simulink model "mitchell_bluetooth"  (R2018b)
settings: Solver=FixedStepDiscrete  StartTime=0.0  StopTime=10.0  FixedStep=0.00005  RelTol=1e-3  EnableMultiTasking=on
libraries: stellaris_lp_lib x13, discretizing x3, etargetslib x1, xpcutilitieslib x1
settings Model: Creator=Mitchell Cassaday  LastModifiedBy=Mitchell Cassaday
settings OptimizationCC: DefaultUnderspecifiedDataType=single  PassReuseOutputArgsAs=Individual arguments  MaxStackSize=64
settings DebuggingCC: BlockPriorityViolationMsg=error  MinStepSizeMsg=error  SolverPrmCheckMsg=warning  MultiTaskRateTransMsg=warning  ParameterTunabilityLossMsg=error
settings HardwareCC: ProdBitPerPointer=32  ProdBitPerSizeT=32  ProdBitPerPtrDiffT=32  ProdLargestAtomicInteger=Long  ProdLargestAtomicFloat=Double  ProdWordSize=32  ProdHWDeviceType=ARM Compatible->ARM Cortex
settings SFSimCC: SimUseLocalCustomCode=off  MATLABDynamicMemAlloc=off
settings RTWCC: SystemTargetFile=ert.tlc  HardwareBoard=Tiva TM4C123G Launchpad  TemplateMakefile=ert_default_tmf  GenerateReport=on  RTWUseLocalCustomCode=off  Toolchain=Texas Instruments Code Composer Studio (Tiva)  BuildConfiguration=Faster Runs  IncludeHyperlinkInReport=on  LaunchReport=on  GenerateTraceInfo=on  GenerateTraceReport=on  GenerateTraceReportSl=on  GenerateTraceReportSf=on  GenerateTraceReportEml=on
settings CodeAppCC: ForceParamTrailComments=on  IgnoreCustomStorageClasses=off  OperatorAnnotations=on  SimulinkDataObjDesc=on  SFDataObjDesc=on  InsertBlockDesc=on

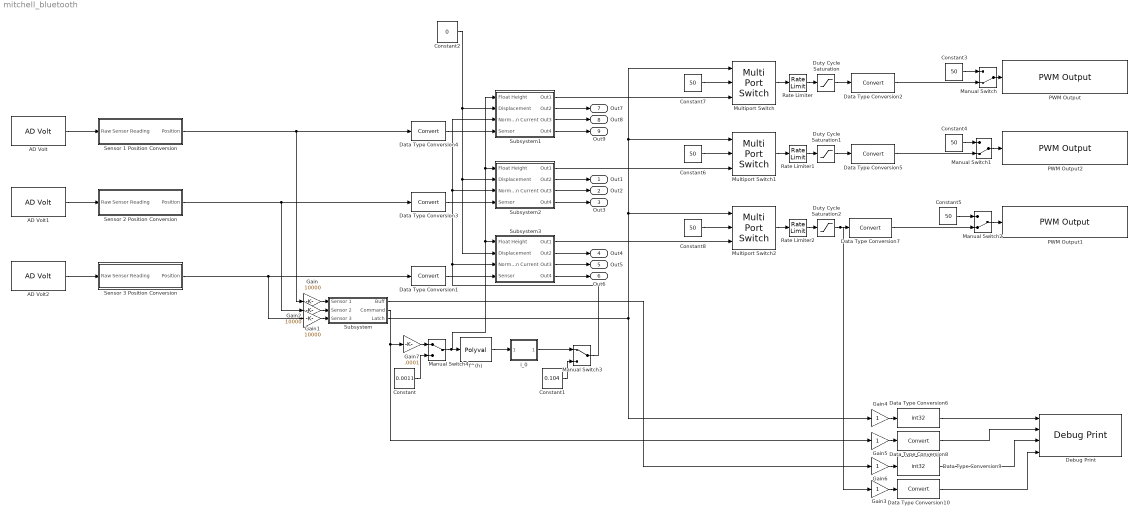
== system mitchell_bluetooth ==
  AD Volt : stellaris_lp_lib/ADC/AD Volt  ch="5   PE5"  sample_time=0.0001
      settings: SourceProductName=Run on Stellaris LaunchPad
  AD Volt1 : stellaris_lp_lib/ADC/AD Volt  ch="3   PE1"  sample_time=0.0001
      settings: SourceProductName=Run on Stellaris LaunchPad
  AD Volt2 : stellaris_lp_lib/ADC/AD Volt  ch="2   PE2"  sample_time=0.0001
      settings: SourceProductName=Run on Stellaris LaunchPad
  Constant : Constant  Value=0.0011
  Constant1 : Constant  Value=0.104
  Constant2 : Constant  Value=0
  Constant{3..8} (6 alike) : Constant  Value=50
  Data Type Conversion{1..5,7..8,10} (8 alike) : DataTypeConversion
  Data Type Conversion6 : DataTypeConversion  OutDataTypeStr=int32
  Data Type Conversion9 : DataTypeConversion  OutDataTypeStr=int32
  Debug Print : stellaris_lp_lib/Debug/Debug Print  fmt="'a: %d    b: %d    c: %d     d:%d'"  sample_time=0.1
      settings: SourceProductName=Run on Stellaris LaunchPad
  Duty Cycle Saturation : Saturate  UpperLimit=99  LowerLimit=0
  Duty Cycle Saturation1 : Saturate  UpperLimit=99  LowerLimit=0
  Duty Cycle Saturation2 : Saturate  UpperLimit=99  LowerLimit=0
  Gain : Gain  Gain=10000
  Gain1 : Gain  Gain=10000
  Gain2 : Gain  Gain=10000
  Gain{3..6} (4 alike) : Gain
  Gain7 : Gain  Gain=.0001
  Manual Switch : ManualSwitch  CurrentSetting=0
  Manual Switch1 : ManualSwitch  CurrentSetting=0
  Manual Switch2 : ManualSwitch  CurrentSetting=0
  Manual Switch3 : ManualSwitch
  Manual Switch4 : ManualSwitch
  Multiport Switch : MultiPortSwitch  DataPortOrder=Zero-based contiguous  Inputs=2  DiagnosticForDefault=None  zeroidx=on
  Multiport Switch1 : MultiPortSwitch  DataPortOrder=Zero-based contiguous  Inputs=2  DiagnosticForDefault=None  zeroidx=on
  Multiport Switch2 : MultiPortSwitch  DataPortOrder=Zero-based contiguous  Inputs=2  DiagnosticForDefault=None  zeroidx=on
  PWM Output : stellaris_lp_lib/PWM/PWM Output  ch="1    PC4"  invert=off  freq=100000  sample_time=-1
      settings: SourceProductName=Run on Stellaris LaunchPad
  PWM Output1 : stellaris_lp_lib/PWM/PWM Output  ch="3    PC6"  invert=off  freq=100000  sample_time=-1
      settings: SourceProductName=Run on Stellaris LaunchPad
  PWM Output2 : stellaris_lp_lib/PWM/PWM Output  ch="2    PC5"  invert=off  freq=100000  sample_time=-1
      settings: SourceProductName=Run on Stellaris LaunchPad
  Rate Limiter : RateLimiter  RisingSlewLimit=10000  FallingSlewLimit=-10000  SampleTimeMode=inherited
  Rate Limiter1 : RateLimiter  RisingSlewLimit=10000  FallingSlewLimit=-10000  SampleTimeMode=inherited
  Rate Limiter2 : RateLimiter  RisingSlewLimit=10000  FallingSlewLimit=-10000  SampleTimeMode=inherited
  Sensor 1 Position Conversion : Subsystem
  Sensor 2 Position Conversion : Subsystem
  Sensor 3 Position Conversion : Subsystem
  Subsystem : Subsystem
  Subsystem1 : Subsystem
  Subsystem2 : Subsystem
  Subsystem3 : Subsystem
  f^(h) : Polyval  Coefs=[ +1.6739e+20, -1.3935e+18, +4.7154e+15, -8.351e+12, +8.2878e+9, -4.527e+6, 1.1593e+3 ]
  "i_0 " : Subsystem
  Out1 : Outport
  Out2 : Outport  Port=2
  Out3 : Outport  Port=3
  Out4 : Outport  Port=4
  Out5 : Outport  Port=5
  Out6 : Outport  Port=6
  Out7 : Outport  Port=7
  Out8 : Outport  Port=8
  Out9 : Outport  Port=9
  wires:
  AD Volt2/1 -> Sensor 3 Position Conversion/1(Raw Sensor Reading)
  AD Volt1/1 -> Sensor 2 Position Conversion/1(Raw Sensor Reading)
  AD Volt/1 -> Sensor 1 Position Conversion/1(Raw Sensor Reading)
  Data Type Conversion3/1 -> Subsystem2/4(Sensor)
  Data Type Conversion4/1 -> Subsystem1/4(Sensor)
  Constant2/1 -> Subsystem1/2(Displacement), Subsystem3/2(Displacement), Subsystem2/2(Displacement)
  Manual Switch3/1 -> Subsystem1/3(Normalization Current), Subsystem2/3(Normalization Current), Subsystem3/3(Normalization Current)
  Manual Switch2/1 -> PWM Output1/1
  Manual Switch1/1 -> PWM Output2/1
  Subsystem2/4(Out4) -> Out3/1
  Data Type Conversion6/1 -> Debug Print/1
  Manual Switch/1 -> PWM Output/1
  Data Type Conversion2/1 -> Manual Switch/2
  Constant3/1 -> Manual Switch/1
  Data Type Conversion5/1 -> Manual Switch1/2
  Constant4/1 -> Manual Switch1/1
  Data Type Conversion7/1 -> Manual Switch2/2
  Constant5/1 -> Manual Switch2/1
  Data Type Conversion8/1 -> Debug Print/2
  Data Type Conversion9/1 -> Debug Print/3
  Data Type Conversion10/1 -> Debug Print/4
  Subsystem2/2(Out2) -> Out1/1
  Subsystem2/3(Out3) -> Out2/1
  Subsystem3/3(Out3) -> Out5/1
  Subsystem3/2(Out2) -> Out4/1
  Subsystem3/4(Out4) -> Out6/1
  Subsystem1/4(Out4) -> Out9/1
  Subsystem1/2(Out2) -> Out7/1
  Subsystem1/3(Out3) -> Out8/1
  Data Type Conversion1/1 -> Subsystem3/4(Sensor)
  Sensor 1 Position Conversion/1(Position) -> Data Type Conversion4/1, Gain/1
  Sensor 2 Position Conversion/1(Position) -> Data Type Conversion3/1, Gain1/1
  Gain/1 -> Subsystem/1("Sensor 1 ")
  Gain1/1 -> Subsystem/2(Sensor 2)
  Gain3/1 -> Data Type Conversion10/1
  Gain2/1 -> Subsystem/3(Sensor 3)
  Gain4/1 -> Data Type Conversion6/1
  Gain5/1 -> Data Type Conversion8/1
  Gain6/1 -> Data Type Conversion9/1
  Sensor 3 Position Conversion/1(Position) -> Data Type Conversion1/1, Gain2/1
  f^(h)/1 -> "i_0 "/1(f^(h0))
  Constant/1 -> Manual Switch4/2
  Constant1/1 -> Manual Switch3/2
  "i_0 "/1(Out1) -> Manual Switch3/1
  Subsystem/1(Buff) -> Gain6/1
  Subsystem1/1(Out1) -> Multiport Switch/3
  Subsystem3/1(Out1) -> Multiport Switch2/3
  Duty Cycle Saturation/1 -> Data Type Conversion2/1
  Duty Cycle Saturation1/1 -> Data Type Conversion5/1
  Duty Cycle Saturation2/1 -> Gain3/1, Data Type Conversion7/1
  Subsystem/2(Command) -> Gain5/1, Gain7/1
  Gain7/1 -> Manual Switch4/1
  Manual Switch4/1 -> f^(h)/1, Subsystem3/1(Float Height), Subsystem2/1(Float Height), Subsystem1/1(Float Height)
  Subsystem/3("Latch ") -> Gain4/1, Multiport Switch/1, Multiport Switch1/1, Multiport Switch2/1
  Multiport Switch/1 -> Rate Limiter/1
  Rate Limiter/1 -> Duty Cycle Saturation/1
  Multiport Switch1/1 -> Rate Limiter1/1
  Rate Limiter1/1 -> Duty Cycle Saturation1/1
  Multiport Switch2/1 -> Rate Limiter2/1
  Rate Limiter2/1 -> Duty Cycle Saturation2/1
  Subsystem2/1(Out1) -> Multiport Switch1/3
  Constant6/1 -> Multiport Switch1/2
  Constant7/1 -> Multiport Switch/2
  Constant8/1 -> Multiport Switch2/2

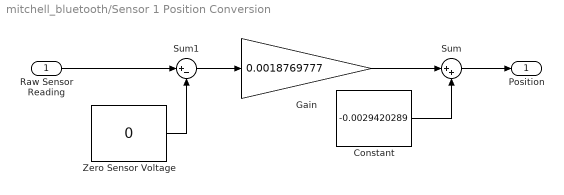
== system mitchell_bluetooth/Sensor 1 Position Conversion ==
  Raw Sensor Reading : Inport
  Constant : Constant  Value=-0.0029420289  OutDataTypeStr=Inherit: Inherit via back propagation
  Gain : Gain  Gain=0.0018769777
  Sum : Sum  Inputs=|++
  Sum1 : Sum  Inputs=|+-
  Zero Sensor Voltage : Constant  Value=0  OutDataTypeStr=Inherit: Inherit via back propagation
  Position : Outport
  wires:
  Gain/1 -> Sum/1
  Constant/1 -> Sum/2
  Sum/1 -> Position/1
  Zero Sensor Voltage/1 -> Sum1/2
  Sum1/1 -> Gain/1
  Raw Sensor Reading/1 -> Sum1/1

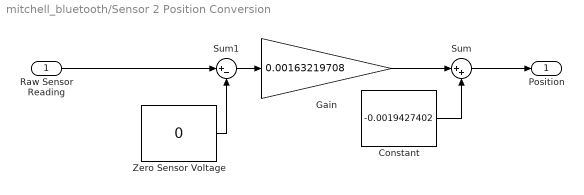
== system mitchell_bluetooth/Sensor 2 Position Conversion ==
  Raw Sensor Reading : Inport
  Constant : Constant  Value=-0.0019427402  OutDataTypeStr=Inherit: Inherit via back propagation
  Gain : Gain  Gain=0.00163219708
  Sum : Sum  Inputs=|++
  Sum1 : Sum  Inputs=|+-
  Zero Sensor Voltage : Constant  Value=0  OutDataTypeStr=Inherit: Inherit via back propagation
  Position : Outport
  wires:
  Gain/1 -> Sum/1
  Constant/1 -> Sum/2
  Sum/1 -> Position/1
  Zero Sensor Voltage/1 -> Sum1/2
  Sum1/1 -> Gain/1
  Raw Sensor Reading/1 -> Sum1/1

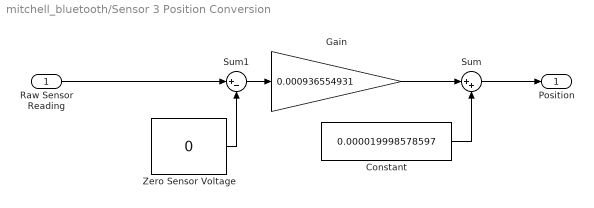
== system mitchell_bluetooth/Sensor 3 Position Conversion ==
  Raw Sensor Reading : Inport
  Constant : Constant  Value=0.000019998578597  OutDataTypeStr=Inherit: Inherit via back propagation
  Gain : Gain  Gain=0.000936554931
  Sum : Sum  Inputs=|++
  Sum1 : Sum  Inputs=|+-
  Zero Sensor Voltage : Constant  Value=0  OutDataTypeStr=Inherit: Inherit via back propagation
  Position : Outport
  wires:
  Gain/1 -> Sum/1
  Constant/1 -> Sum/2
  Sum/1 -> Position/1
  Zero Sensor Voltage/1 -> Sum1/2
  Sum1/1 -> Gain/1
  Raw Sensor Reading/1 -> Sum1/1

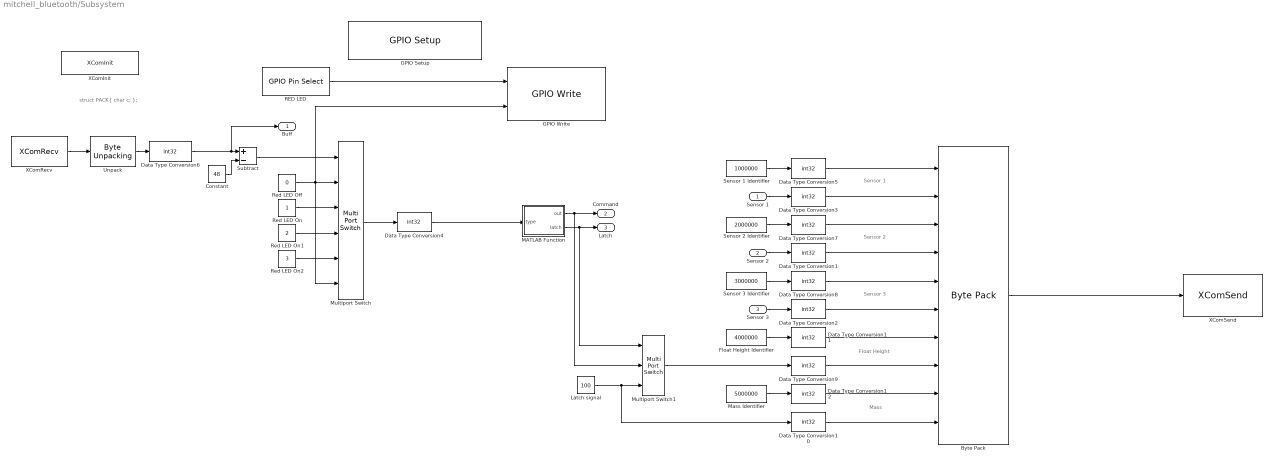
== system mitchell_bluetooth/Subsystem ==
  note: Sensor 1
  note: struct  PACK{
      | 		char c;
      | };
  note: Sensor 2
  note: Sensor 3
  note: Float Height
  note: Mass
  "Sensor 1 " : Inport
  Sensor 2 : Inport  Port=2
  Sensor 3 : Inport  Port=3
  Byte Pack : etargetslib/Byte Pack  datatypes={'int32','int32','int32','int32','int32','int32','int32','int32','int32','int32'}  byteAlign=1
  Constant : Constant  Value=48  OutDataTypeStr=int32
  Data Type Conversion{1..12} (12 alike) : DataTypeConversion  OutDataTypeStr=int32
  Float Height Identifier : Constant  Value=4000000  OutDataTypeStr=int32
  GPIO Setup : stellaris_lp_lib/GPIO/GPIO Setup  GPIO_PORTX_BASE=GPIO_PORTF_BASE  PinsOutput_0=Input  PinsOutput_1=Output  PinsOutput_2=Output  PinsOutput_3=Output  PinsOutput_4=Input  PinsOutput_5=Input  PinsOutput_6=Input  PinsOutput_7=Input
      settings: SourceProductName=Run on Stellaris LaunchPad
  GPIO Write : stellaris_lp_lib/GPIO/GPIO Write  GPIO_PORTX_BASE=GPIO_PORTF_BASE  SampleTime=-1
      settings: SourceProductName=Run on Stellaris LaunchPad
  Latch signal : Constant  Value=100  OutDataTypeStr=uint8
  MATLAB Function : MATLAB Function  TreatAsAtomicUnit=on
  Mass Identifier : Constant  Value=5000000  OutDataTypeStr=int32
  Multiport Switch : MultiPortSwitch  DataPortOrder=Zero-based contiguous  Inputs=5  DiagnosticForDefault=None  zeroidx=on
  Multiport Switch1 : MultiPortSwitch  DataPortOrder=Zero-based contiguous  Inputs=2  DiagnosticForDefault=None  zeroidx=on
  RED LED : stellaris_lp_lib/GPIO/GPIO Pin Select  GPIO_PIN_X=GPIO_PIN_1
      settings: SourceProductName=Run on Stellaris LaunchPad
  Red LED Off : Constant  Value=0  OutDataTypeStr=uint8
  Red LED On : Constant  OutDataTypeStr=uint8
  Red LED On1 : Constant  Value=2  OutDataTypeStr=uint8
  Red LED On2 : Constant  Value=3  OutDataTypeStr=uint8
  Sensor 1 Identifier : Constant  Value=1000000  OutDataTypeStr=int32
  Sensor 2 Identifier : Constant  Value=2000000  OutDataTypeStr=int32
  Sensor 3 Identifier : Constant  Value=3000000  OutDataTypeStr=int32
  Subtract : Sum  Inputs=+-
  Unpack : xpcutilitieslib/Byte Unpacking   MaskUnpackedDataTypes={'uint8'}  MaskUnpackedDataSizes={1}  MaskAlignment=1
      settings: SourceProductName=Simulink Real-Time  SourceProductBaseCode=XP
  XComInit : stellaris_lp_lib/Communication/XComInit  baud=9600
      settings: SourceProductName=Run on Stellaris LaunchPad
  XComRecv : stellaris_lp_lib/Communication/XComRecv  pack_size=1  sample_time=.001
      settings: SourceProductName=Run on Stellaris LaunchPad
  XComSend : stellaris_lp_lib/Communication/XComSend  pack_size=40  sample_time=0.1
      settings: SourceProductName=Run on Stellaris LaunchPad
  Buff : Outport
  Command : Outport  Port=2
  "Latch " : Outport  Port=3
  wires:
  XComRecv/1 -> Unpack/1
  Unpack/1 -> Data Type Conversion6/1
  Byte Pack/1 -> XComSend/1
  Red LED On/1 -> Multiport Switch/3
  "Sensor 1 "/1 -> Data Type Conversion3/1
  Constant/1 -> Subtract/2
  Red LED Off/1 -> Multiport Switch/6, GPIO Write/2, Multiport Switch/2
  RED LED/1 -> GPIO Write/1
  Sensor 2/1 -> Data Type Conversion1/1
  Sensor 3/1 -> Data Type Conversion2/1
  MATLAB Function/1(out) -> Command/1, Multiport Switch1/2
  Subtract/1 -> Multiport Switch/1
  Multiport Switch/1 -> Data Type Conversion4/1
  Red LED On1/1 -> Multiport Switch/4
  Red LED On2/1 -> Multiport Switch/5
  Data Type Conversion4/1 -> MATLAB Function/1(type)
  MATLAB Function/2(latch) -> Multiport Switch1/1, "Latch "/1
  Data Type Conversion6/1 -> Subtract/1, Buff/1
  Sensor 1 Identifier/1 -> Data Type Conversion5/1
  Data Type Conversion1/1 -> Byte Pack/4
  Sensor 2 Identifier/1 -> Data Type Conversion7/1
  Data Type Conversion3/1 -> Byte Pack/2
  Sensor 3 Identifier/1 -> Data Type Conversion8/1
  Data Type Conversion2/1 -> Byte Pack/6
  Data Type Conversion5/1 -> Byte Pack/1
  Data Type Conversion7/1 -> Byte Pack/3
  Data Type Conversion8/1 -> Byte Pack/5
  Data Type Conversion11/1 -> Byte Pack/7
  Data Type Conversion9/1 -> Byte Pack/8
  Data Type Conversion12/1 -> Byte Pack/9
  Data Type Conversion10/1 -> Byte Pack/10
  Float Height Identifier/1 -> Data Type Conversion11/1
  Mass Identifier/1 -> Data Type Conversion12/1
  Latch signal/1 -> Data Type Conversion10/1, Multiport Switch1/3
  Multiport Switch1/1 -> Data Type Conversion9/1

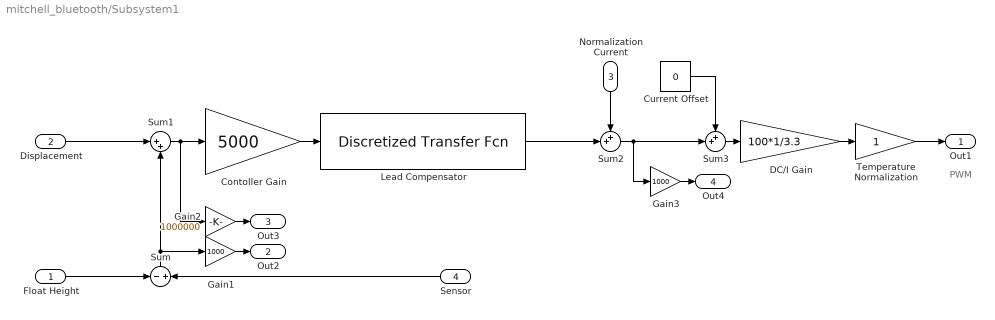
== system mitchell_bluetooth/Subsystem1 ==
  note: PWM
  Float Height : Inport
  Displacement : Inport  Port=2
  Normalization Current : Inport  Port=3
  Sensor : Inport  Port=4
  Contoller Gain : Gain  Gain=5000
  Current Offset : Constant  Value=0
  DC/I Gain : Gain  Gain=100*1/3.3
  Gain1 : Gain  Gain=1000
  Gain2 : Gain  Gain=1000000
  Gain3 : Gain  Gain=1000
  Lead Compensator : discretizing/Discretized Transfer Fcn  Numerator=[1 550]  Denominator=[1 3100]  AbsTol=auto  SampleTime=0.0001  method=zoh  Wc=0
  Sum : Sum  Inputs=-|+
  Sum1 : Sum  Inputs=|++
  Sum2 : Sum  Inputs=++|
  Sum3 : Sum  Inputs=++|
  Temperature Normalization : Gain
  Out1 : Outport  OutMin=[0]  OutMax=[100]
  Out2 : Outport  Port=2
  Out3 : Outport  Port=3
  Out4 : Outport  Port=4
  wires:
  Gain3/1 -> Out4/1
  Sum/1 -> Gain1/1, Sum1/2
  Contoller Gain/1 -> Lead Compensator/1
  Lead Compensator/1 -> Sum2/2
  Sum2/1 -> Sum3/2, Gain3/1
  Gain1/1 -> Out2/1
  Float Height/1 -> Sum/1
  Temperature Normalization/1 -> Out1/1
  Gain2/1 -> Out3/1
  Sensor/1 -> Sum/2
  Sum1/1 -> Gain2/1, Contoller Gain/1
  Displacement/1 -> Sum1/1
  Normalization Current/1 -> Sum2/1
  Sum3/1 -> DC/I Gain/1
  DC/I Gain/1 -> Temperature Normalization/1
  Current Offset/1 -> Sum3/1

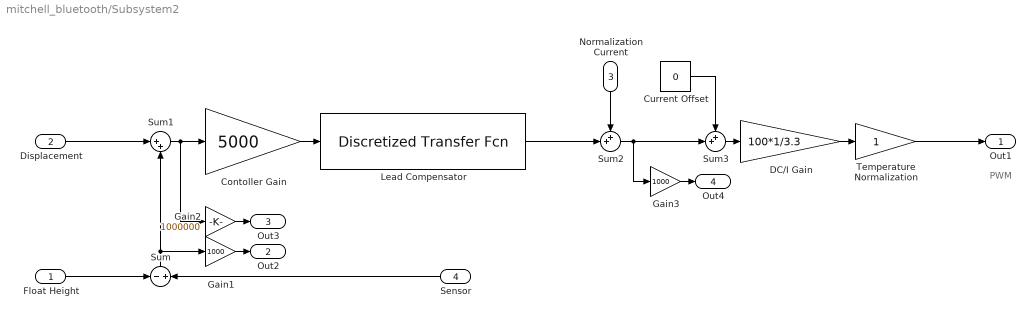
== system mitchell_bluetooth/Subsystem2 ==
  note: PWM
  Float Height : Inport
  Displacement : Inport  Port=2
  Normalization Current : Inport  Port=3
  Sensor : Inport  Port=4
  Contoller Gain : Gain  Gain=5000
  Current Offset : Constant  Value=0
  DC/I Gain : Gain  Gain=100*1/3.3
  Gain1 : Gain  Gain=1000
  Gain2 : Gain  Gain=1000000
  Gain3 : Gain  Gain=1000
  Lead Compensator : discretizing/Discretized Transfer Fcn  Numerator=[1 550]  Denominator=[1 3100]  AbsTol=auto  SampleTime=0.0001  method=zoh  Wc=0
  Sum : Sum  Inputs=-|+
  Sum1 : Sum  Inputs=|++
  Sum2 : Sum  Inputs=++|
  Sum3 : Sum  Inputs=++|
  Temperature Normalization : Gain
  Out1 : Outport  OutMin=[0]  OutMax=[100]
  Out2 : Outport  Port=2
  Out3 : Outport  Port=3
  Out4 : Outport  Port=4
  wires:
  Gain3/1 -> Out4/1
  Sum/1 -> Gain1/1, Sum1/2
  Contoller Gain/1 -> Lead Compensator/1
  Lead Compensator/1 -> Sum2/2
  Sum2/1 -> Sum3/2, Gain3/1
  Gain1/1 -> Out2/1
  Float Height/1 -> Sum/1
  Temperature Normalization/1 -> Out1/1
  Gain2/1 -> Out3/1
  Sensor/1 -> Sum/2
  Sum1/1 -> Gain2/1, Contoller Gain/1
  Displacement/1 -> Sum1/1
  Normalization Current/1 -> Sum2/1
  Sum3/1 -> DC/I Gain/1
  DC/I Gain/1 -> Temperature Normalization/1
  Current Offset/1 -> Sum3/1

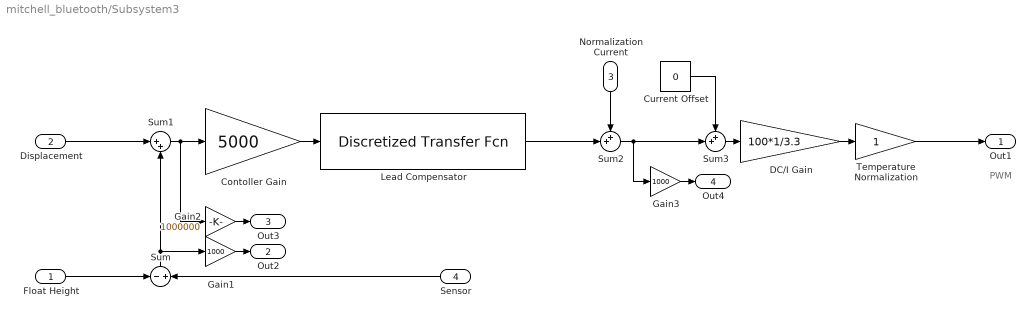
== system mitchell_bluetooth/Subsystem3 ==
  note: PWM
  Float Height : Inport
  Displacement : Inport  Port=2
  Normalization Current : Inport  Port=3
  Sensor : Inport  Port=4
  Contoller Gain : Gain  Gain=5000
  Current Offset : Constant  Value=0
  DC/I Gain : Gain  Gain=100*1/3.3
  Gain1 : Gain  Gain=1000
  Gain2 : Gain  Gain=1000000
  Gain3 : Gain  Gain=1000
  Lead Compensator : discretizing/Discretized Transfer Fcn  Numerator=[1 550]  Denominator=[1 3100]  AbsTol=auto  SampleTime=0.0001  method=zoh  Wc=0
  Sum : Sum  Inputs=-|+
  Sum1 : Sum  Inputs=|++
  Sum2 : Sum  Inputs=++|
  Sum3 : Sum  Inputs=++|
  Temperature Normalization : Gain
  Out1 : Outport  OutMin=[0]  OutMax=[100]
  Out2 : Outport  Port=2
  Out3 : Outport  Port=3
  Out4 : Outport  Port=4
  wires:
  Gain3/1 -> Out4/1
  Sum/1 -> Gain1/1, Sum1/2
  Contoller Gain/1 -> Lead Compensator/1
  Lead Compensator/1 -> Sum2/2
  Sum2/1 -> Sum3/2, Gain3/1
  Gain1/1 -> Out2/1
  Float Height/1 -> Sum/1
  Temperature Normalization/1 -> Out1/1
  Gain2/1 -> Out3/1
  Sensor/1 -> Sum/2
  Sum1/1 -> Gain2/1, Contoller Gain/1
  Displacement/1 -> Sum1/1
  Normalization Current/1 -> Sum2/1
  Sum3/1 -> DC/I Gain/1
  DC/I Gain/1 -> Temperature Normalization/1
  Current Offset/1 -> Sum3/1

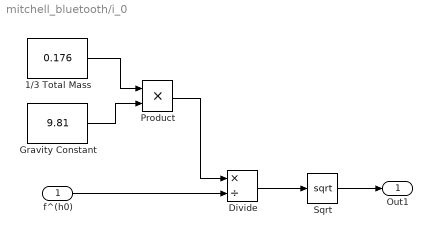
== system mitchell_bluetooth/i_0  ==
  f^(h0) : Inport
  1/3 Total Mass : Constant  Value=0.176
  Divide : Product  Inputs=*/
  Gravity Constant : Constant  Value=9.81
  Product : Product
  Sqrt : Sqrt  SaturateOnIntegerOverflow=on
  Out1 : Outport
  wires:
  1/3 Total Mass/1 -> Product/1
  Gravity Constant/1 -> Product/2
  Sqrt/1 -> Out1/1
  Product/1 -> Divide/1
  f^(h0)/1 -> Divide/2
  Divide/1 -> Sqrt/1

== matlab function mitchell_bluetooth/Subsystem/MATLAB Function ==
  data: type input; out output; latch output
function [out, latch]= fcn(type)
    persistent val;
    persistent output;
    persistent hold;
    persistent latched;
    if isempty(val)
        val = cast(0,'int32');
        output = 9;
        hold = 0;
    end
    if isempty(latched)
        latched = cast(1, 'int32');
    end
    if type == 0 
        if val == 1
            output = output + 1;
        elseif val == 2
            output = output - 1;
        elseif val == 3
%             if not(latched)
%                 hold = output;
%                 output = 0;
%             else
%                 output = hold;
%             end
            latched = cast(not(latched), 'int32');
        end
        val = cast(0,'int32');
    elseif type > 0
        val = type;
    end
    out = output;
    latch = latched;
